simulink subsystem "tcp_trace_simscape_ref_subsys"  (R2022b)
settings: Solver=VariableStepAuto  StartTime=0.0  StopTime=10.0  RelTol=1e-3
undefined symbols (not defined in the file): param_vis
libraries: nesl_utility x300, sm_lib x200
(part 2 of 3)

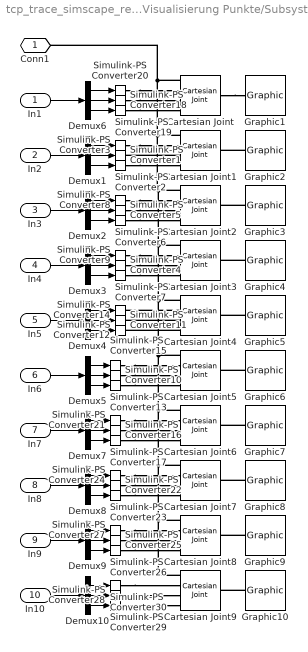
== system tcp_trace_simscape_ref_subsys/Visualisierung Punkte/Subsystem3 ==
  In1 : Inport
  In2 : Inport  Port=2
  In3 : Inport  Port=3
  In4 : Inport  Port=4
  In5 : Inport  Port=5
  In6 : Inport  Port=6
  In7 : Inport  Port=7
  In8 : Inport  Port=8
  In9 : Inport  Port=9
  In10 : Inport  Port=10
  Cartesian Joint{,1..9} (10 alike) : sm_lib/Joints/Cartesian Joint  JointMode=Normal  SenseConstraintForce=off  SenseConstraintForceX=off  SenseConstraintForceY=off  SenseConstraintForceZ=off  SenseConstraintTorque=off  SenseConstraintTorqueX=off  SenseConstraintTorqueY=off  SenseConstraintTorqueZ=off  SenseTotalForce=off  SenseTotalForceX=off  SenseTotalForceY=off  SenseTotalForceZ=off  SenseTotalTorque=off  SenseTotalTorqueX=off  SenseTotalTorqueY=off  SenseTotalTorqueZ=off  CompositeWrenchDir=FollowerOnBase  CompositeWrenchFrame=BaseFrame  PxEquilibriumPosition=0  PxEquilibriumPositionUnits=m  PxSpringStiffness=0  PxSpringStiffnessUnits=N/m  PxDampingCoefficient=0  PxDampingCoefficientUnits=N/(m/s)  PxTorqueActuationMode=ComputedTorque  PxMotionActuationMode=InputMotion  PxSensePosition=off  PxSenseVelocity=off  PxSenseAcceleration=off  PxSenseTorqueForce=off  PxSenseLowerLimitTorqueForce=off  PxSenseUpperLimitTorqueForce=off  PxLowerLimitSpecify=off  PxLowerLimitBound=-1  PxLowerLimitBoundUnits=m  PxLowerLimitStiffness=1e6  PxLowerLimitStiffnessUnits=N/m  PxLowerLimitDamping=1e3  PxLowerLimitDampingUnits=N/(m/s)  PxLowerLimitTransitionRegionWidth=1e-4  PxLowerLimitTransitionRegionWidthUnits=m  PxUpperLimitSpecify=off  PxUpperLimitBound=1  PxUpperLimitBoundUnits=m  PxUpperLimitStiffness=1e6  PxUpperLimitStiffnessUnits=N/m  PxUpperLimitDamping=1e3  PxUpperLimitDampingUnits=N/(m/s)  PxUpperLimitTransitionRegionWidth=1e-4  PxUpperLimitTransitionRegionWidthUnits=m  PxPositionTargetSpecify=off  PxPositionTargetPriority=High  PxPositionTargetValue=0  PxPositionTargetValueUnits=m  PxVelocityTargetSpecify=off  PxVelocityTargetPriority=High  PxVelocityTargetValue=0  PxVelocityTargetValueUnits=m/s  PyEquilibriumPosition=0  PyEquilibriumPositionUnits=m  PySpringStiffness=0  PySpringStiffnessUnits=N/m  PyDampingCoefficient=0  PyDampingCoefficientUnits=N/(m/s)  PyTorqueActuationMode=ComputedTorque  PyMotionActuationMode=InputMotion  PySensePosition=off  PySenseVelocity=off  PySenseAcceleration=off  PySenseTorqueForce=off  PySenseLowerLimitTorqueForce=off  PySenseUpperLimitTorqueForce=off  PyLowerLimitSpecify=off  PyLowerLimitBound=-1  PyLowerLimitBoundUnits=m  PyLowerLimitStiffness=1e6  PyLowerLimitStiffnessUnits=N/m  PyLowerLimitDamping=1e3  PyLowerLimitDampingUnits=N/(m/s)  PyLowerLimitTransitionRegionWidth=1e-4  PyLowerLimitTransitionRegionWidthUnits=m  PyUpperLimitSpecify=off  PyUpperLimitBound=1  PyUpperLimitBoundUnits=m  PyUpperLimitStiffness=1e6  PyUpperLimitStiffnessUnits=N/m  PyUpperLimitDamping=1e3  PyUpperLimitDampingUnits=N/(m/s)  PyUpperLimitTransitionRegionWidth=1e-4  PyUpperLimitTransitionRegionWidthUnits=m  PyPositionTargetSpecify=off  PyPositionTargetPriority=High  PyPositionTargetValue=0  PyPositionTargetValueUnits=m  PyVelocityTargetSpecify=off  PyVelocityTargetPriority=High  PyVelocityTargetValue=0  PyVelocityTargetValueUnits=m/s  PzEquilibriumPosition=0  PzEquilibriumPositionUnits=m  PzSpringStiffness=0  PzSpringStiffnessUnits=N/m  PzDampingCoefficient=0  PzDampingCoefficientUnits=N/(m/s)  PzTorqueActuationMode=ComputedTorque  PzMotionActuationMode=InputMotion  PzSensePosition=off  PzSenseVelocity=off  PzSenseAcceleration=off  PzSenseTorqueForce=off  PzSenseLowerLimitTorqueForce=off  PzSenseUpperLimitTorqueForce=off  PzLowerLimitSpecify=off  PzLowerLimitBound=-1  PzLowerLimitBoundUnits=m  PzLowerLimitStiffness=1e6  PzLowerLimitStiffnessUnits=N/m  PzLowerLimitDamping=1e3  PzLowerLimitDampingUnits=N/(m/s)  PzLowerLimitTransitionRegionWidth=1e-4  PzLowerLimitTransitionRegionWidthUnits=m  PzUpperLimitSpecify=off  PzUpperLimitBound=1  PzUpperLimitBoundUnits=m  PzUpperLimitStiffness=1e6  PzUpperLimitStiffnessUnits=N/m  PzUpperLimitDamping=1e3  PzUpperLimitDampingUnits=N/(m/s)  PzUpperLimitTransitionRegionWidth=1e-4  PzUpperLimitTransitionRegionWidthUnits=m  PzPositionTargetSpecify=off  PzPositionTargetPriority=High  PzPositionTargetValue=0  PzPositionTargetValueUnits=m  PzVelocityTargetSpecify=off  PzVelocityTargetPriority=High  PzVelocityTargetValue=0  PzVelocityTargetValueUnits=m/s
  Demux{1..10} (10 alike) : Demux  Outputs=3
  Graphic{1..10} (10 alike) : sm_lib/Body Elements/Graphic  GraphicType=Marker  MarkerShape=Sphere  MarkerSize=param_vis.vis_point.pix  GraphicVisPropType=SimpleVisualProperties  GraphicDiffuseColor=param_vis.vis_point.col  GraphicSpecularColor=[0.5 0.5 0.5 1.0]  GraphicAmbientColor=[0.15 0.15 0.15 1.0]  GraphicEmissiveColor=[0.0 0.0 0.0 1.0]  GraphicShininess=75  GraphicOpacity=param_vis.vis_point.opa
  Simulink-PS Converter{1..30} (30 alike) : nesl_utility/Simulink-PS Converter  PhysicalDomain=network_engine_domain  SubClassName=ps_input  LeftPortType=input  RightPortType=output  PseudoPeriodic=off  Frequencies=[]  NoiseDistribution=none  NoiseParameters=[]  Unit=1  AffineConversion=off  FilteringAndDerivatives=zero  SimscapeFilterOrder=2  InputFilterTimeConstant=0.001  UdotUserProvided=0
  Conn1 : PMIOPort  Side=Left
  wires:
  Demux10/3 -> Simulink-PS Converter29/1
  Demux10/2 -> Simulink-PS Converter28/1
  Demux10/1 -> Simulink-PS Converter30/1
  Demux9/3 -> Simulink-PS Converter26/1
  Demux9/2 -> Simulink-PS Converter25/1
  Demux9/1 -> Simulink-PS Converter27/1
  Demux8/3 -> Simulink-PS Converter23/1
  Demux8/2 -> Simulink-PS Converter22/1
  Demux8/1 -> Simulink-PS Converter24/1
  Demux7/3 -> Simulink-PS Converter17/1
  Demux7/2 -> Simulink-PS Converter16/1
  Demux7/1 -> Simulink-PS Converter21/1
  Demux5/3 -> Simulink-PS Converter13/1
  Demux5/2 -> Simulink-PS Converter10/1
  Demux5/1 -> Simulink-PS Converter15/1
  Demux3/2 -> Simulink-PS Converter4/1
  Demux3/1 -> Simulink-PS Converter9/1
  Demux3/3 -> Simulink-PS Converter7/1
  Demux2/3 -> Simulink-PS Converter6/1
  Demux2/2 -> Simulink-PS Converter5/1
  Demux2/1 -> Simulink-PS Converter8/1
  Demux1/3 -> Simulink-PS Converter2/1
  Demux1/2 -> Simulink-PS Converter1/1
  Demux4/3 -> Simulink-PS Converter12/1
  Demux4/1 -> Simulink-PS Converter14/1
  Demux4/2 -> Simulink-PS Converter11/1
  Demux1/1 -> Simulink-PS Converter3/1
  Demux6/2 -> Simulink-PS Converter18/1
  Demux6/1 -> Simulink-PS Converter20/1
  In8/1 -> Demux8/1
  In9/1 -> Demux9/1
  In1/1 -> Demux6/1
  In3/1 -> Demux2/1
  Demux6/3 -> Simulink-PS Converter19/1
  In4/1 -> Demux3/1
  In5/1 -> Demux4/1
  In2/1 -> Demux1/1
  In10/1 -> Demux10/1
  In6/1 -> Demux5/1
  In7/1 -> Demux7/1
  connections:
  Simulink-PS Converter7/RConn1 -- Cartesian Joint3/LConn4
  Simulink-PS Converter4/RConn1 -- Cartesian Joint3/LConn3
  Simulink-PS Converter9/RConn1 -- Cartesian Joint3/LConn2
  Simulink-PS Converter29/RConn1 -- Cartesian Joint9/LConn4
  Simulink-PS Converter28/RConn1 -- Cartesian Joint9/LConn3
  Simulink-PS Converter30/RConn1 -- Cartesian Joint9/LConn2
  Simulink-PS Converter26/RConn1 -- Cartesian Joint8/LConn4
  Simulink-PS Converter25/RConn1 -- Cartesian Joint8/LConn3
  Simulink-PS Converter27/RConn1 -- Cartesian Joint8/LConn2
  Simulink-PS Converter23/RConn1 -- Cartesian Joint7/LConn4
  Simulink-PS Converter22/RConn1 -- Cartesian Joint7/LConn3
  Simulink-PS Converter24/RConn1 -- Cartesian Joint7/LConn2
  Simulink-PS Converter17/RConn1 -- Cartesian Joint6/LConn4
  Simulink-PS Converter16/RConn1 -- Cartesian Joint6/LConn3
  Simulink-PS Converter21/RConn1 -- Cartesian Joint6/LConn2
  Simulink-PS Converter13/RConn1 -- Cartesian Joint5/LConn4
  Simulink-PS Converter10/RConn1 -- Cartesian Joint5/LConn3
  Simulink-PS Converter15/RConn1 -- Cartesian Joint5/LConn2
  Simulink-PS Converter2/RConn1 -- Cartesian Joint1/LConn4
  Cartesian Joint1/LConn3 -- Simulink-PS Converter1/RConn1
  Simulink-PS Converter3/RConn1 -- Cartesian Joint1/LConn2
  Cartesian Joint4/LConn3 -- Simulink-PS Converter11/RConn1
  Cartesian Joint4/LConn2 -- Simulink-PS Converter14/RConn1
  Cartesian Joint4/LConn4 -- Simulink-PS Converter12/RConn1
  Simulink-PS Converter5/RConn1 -- Cartesian Joint2/LConn3
  Simulink-PS Converter8/RConn1 -- Cartesian Joint2/LConn2
  Simulink-PS Converter6/RConn1 -- Cartesian Joint2/LConn4
  Simulink-PS Converter20/RConn1 -- Cartesian Joint/LConn2
  Simulink-PS Converter18/RConn1 -- Cartesian Joint/LConn3
  Graphic10/RConn1 -- Cartesian Joint9/RConn1
  Graphic5/RConn1 -- Cartesian Joint4/RConn1
  Graphic2/RConn1 -- Cartesian Joint1/RConn1
  Graphic9/RConn1 -- Cartesian Joint8/RConn1
  Graphic6/RConn1 -- Cartesian Joint5/RConn1
  Graphic8/RConn1 -- Cartesian Joint7/RConn1
  Graphic7/RConn1 -- Cartesian Joint6/RConn1
  Conn1/RConn1 -- Cartesian Joint/LConn1 -- Cartesian Joint1/LConn1 -- Cartesian Joint2/LConn1 -- Cartesian Joint3/LConn1 -- Cartesian Joint4/LConn1 -- Cartesian Joint5/LConn1 -- Cartesian Joint6/LConn1 -- Cartesian Joint7/LConn1 -- Cartesian Joint9/LConn1 -- Cartesian Joint8/LConn1
  Graphic3/RConn1 -- Cartesian Joint2/RConn1
  Cartesian Joint/RConn1 -- Graphic1/RConn1
  Graphic4/RConn1 -- Cartesian Joint3/RConn1
  Simulink-PS Converter19/RConn1 -- Cartesian Joint/LConn4

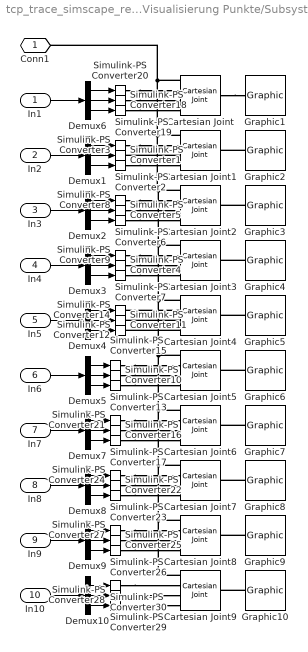
== system tcp_trace_simscape_ref_subsys/Visualisierung Punkte/Subsystem4 ==
  In1 : Inport
  In2 : Inport  Port=2
  In3 : Inport  Port=3
  In4 : Inport  Port=4
  In5 : Inport  Port=5
  In6 : Inport  Port=6
  In7 : Inport  Port=7
  In8 : Inport  Port=8
  In9 : Inport  Port=9
  In10 : Inport  Port=10
  Cartesian Joint{,1..9} (10 alike) : sm_lib/Joints/Cartesian Joint  JointMode=Normal  SenseConstraintForce=off  SenseConstraintForceX=off  SenseConstraintForceY=off  SenseConstraintForceZ=off  SenseConstraintTorque=off  SenseConstraintTorqueX=off  SenseConstraintTorqueY=off  SenseConstraintTorqueZ=off  SenseTotalForce=off  SenseTotalForceX=off  SenseTotalForceY=off  SenseTotalForceZ=off  SenseTotalTorque=off  SenseTotalTorqueX=off  SenseTotalTorqueY=off  SenseTotalTorqueZ=off  CompositeWrenchDir=FollowerOnBase  CompositeWrenchFrame=BaseFrame  PxEquilibriumPosition=0  PxEquilibriumPositionUnits=m  PxSpringStiffness=0  PxSpringStiffnessUnits=N/m  PxDampingCoefficient=0  PxDampingCoefficientUnits=N/(m/s)  PxTorqueActuationMode=ComputedTorque  PxMotionActuationMode=InputMotion  PxSensePosition=off  PxSenseVelocity=off  PxSenseAcceleration=off  PxSenseTorqueForce=off  PxSenseLowerLimitTorqueForce=off  PxSenseUpperLimitTorqueForce=off  PxLowerLimitSpecify=off  PxLowerLimitBound=-1  PxLowerLimitBoundUnits=m  PxLowerLimitStiffness=1e6  PxLowerLimitStiffnessUnits=N/m  PxLowerLimitDamping=1e3  PxLowerLimitDampingUnits=N/(m/s)  PxLowerLimitTransitionRegionWidth=1e-4  PxLowerLimitTransitionRegionWidthUnits=m  PxUpperLimitSpecify=off  PxUpperLimitBound=1  PxUpperLimitBoundUnits=m  PxUpperLimitStiffness=1e6  PxUpperLimitStiffnessUnits=N/m  PxUpperLimitDamping=1e3  PxUpperLimitDampingUnits=N/(m/s)  PxUpperLimitTransitionRegionWidth=1e-4  PxUpperLimitTransitionRegionWidthUnits=m  PxPositionTargetSpecify=off  PxPositionTargetPriority=High  PxPositionTargetValue=0  PxPositionTargetValueUnits=m  PxVelocityTargetSpecify=off  PxVelocityTargetPriority=High  PxVelocityTargetValue=0  PxVelocityTargetValueUnits=m/s  PyEquilibriumPosition=0  PyEquilibriumPositionUnits=m  PySpringStiffness=0  PySpringStiffnessUnits=N/m  PyDampingCoefficient=0  PyDampingCoefficientUnits=N/(m/s)  PyTorqueActuationMode=ComputedTorque  PyMotionActuationMode=InputMotion  PySensePosition=off  PySenseVelocity=off  PySenseAcceleration=off  PySenseTorqueForce=off  PySenseLowerLimitTorqueForce=off  PySenseUpperLimitTorqueForce=off  PyLowerLimitSpecify=off  PyLowerLimitBound=-1  PyLowerLimitBoundUnits=m  PyLowerLimitStiffness=1e6  PyLowerLimitStiffnessUnits=N/m  PyLowerLimitDamping=1e3  PyLowerLimitDampingUnits=N/(m/s)  PyLowerLimitTransitionRegionWidth=1e-4  PyLowerLimitTransitionRegionWidthUnits=m  PyUpperLimitSpecify=off  PyUpperLimitBound=1  PyUpperLimitBoundUnits=m  PyUpperLimitStiffness=1e6  PyUpperLimitStiffnessUnits=N/m  PyUpperLimitDamping=1e3  PyUpperLimitDampingUnits=N/(m/s)  PyUpperLimitTransitionRegionWidth=1e-4  PyUpperLimitTransitionRegionWidthUnits=m  PyPositionTargetSpecify=off  PyPositionTargetPriority=High  PyPositionTargetValue=0  PyPositionTargetValueUnits=m  PyVelocityTargetSpecify=off  PyVelocityTargetPriority=High  PyVelocityTargetValue=0  PyVelocityTargetValueUnits=m/s  PzEquilibriumPosition=0  PzEquilibriumPositionUnits=m  PzSpringStiffness=0  PzSpringStiffnessUnits=N/m  PzDampingCoefficient=0  PzDampingCoefficientUnits=N/(m/s)  PzTorqueActuationMode=ComputedTorque  PzMotionActuationMode=InputMotion  PzSensePosition=off  PzSenseVelocity=off  PzSenseAcceleration=off  PzSenseTorqueForce=off  PzSenseLowerLimitTorqueForce=off  PzSenseUpperLimitTorqueForce=off  PzLowerLimitSpecify=off  PzLowerLimitBound=-1  PzLowerLimitBoundUnits=m  PzLowerLimitStiffness=1e6  PzLowerLimitStiffnessUnits=N/m  PzLowerLimitDamping=1e3  PzLowerLimitDampingUnits=N/(m/s)  PzLowerLimitTransitionRegionWidth=1e-4  PzLowerLimitTransitionRegionWidthUnits=m  PzUpperLimitSpecify=off  PzUpperLimitBound=1  PzUpperLimitBoundUnits=m  PzUpperLimitStiffness=1e6  PzUpperLimitStiffnessUnits=N/m  PzUpperLimitDamping=1e3  PzUpperLimitDampingUnits=N/(m/s)  PzUpperLimitTransitionRegionWidth=1e-4  PzUpperLimitTransitionRegionWidthUnits=m  PzPositionTargetSpecify=off  PzPositionTargetPriority=High  PzPositionTargetValue=0  PzPositionTargetValueUnits=m  PzVelocityTargetSpecify=off  PzVelocityTargetPriority=High  PzVelocityTargetValue=0  PzVelocityTargetValueUnits=m/s
  Demux{1..10} (10 alike) : Demux  Outputs=3
  Graphic{1..10} (10 alike) : sm_lib/Body Elements/Graphic  GraphicType=Marker  MarkerShape=Sphere  MarkerSize=param_vis.vis_point.pix  GraphicVisPropType=SimpleVisualProperties  GraphicDiffuseColor=param_vis.vis_point.col  GraphicSpecularColor=[0.5 0.5 0.5 1.0]  GraphicAmbientColor=[0.15 0.15 0.15 1.0]  GraphicEmissiveColor=[0.0 0.0 0.0 1.0]  GraphicShininess=75  GraphicOpacity=param_vis.vis_point.opa
  Simulink-PS Converter{1..30} (30 alike) : nesl_utility/Simulink-PS Converter  PhysicalDomain=network_engine_domain  SubClassName=ps_input  LeftPortType=input  RightPortType=output  PseudoPeriodic=off  Frequencies=[]  NoiseDistribution=none  NoiseParameters=[]  Unit=1  AffineConversion=off  FilteringAndDerivatives=zero  SimscapeFilterOrder=2  InputFilterTimeConstant=0.001  UdotUserProvided=0
  Conn1 : PMIOPort  Side=Left
  wires:
  In7/1 -> Demux7/1
  In6/1 -> Demux5/1
  In10/1 -> Demux10/1
  In2/1 -> Demux1/1
  In5/1 -> Demux4/1
  In4/1 -> Demux3/1
  Demux6/3 -> Simulink-PS Converter19/1
  In3/1 -> Demux2/1
  In1/1 -> Demux6/1
  In9/1 -> Demux9/1
  In8/1 -> Demux8/1
  Demux6/1 -> Simulink-PS Converter20/1
  Demux6/2 -> Simulink-PS Converter18/1
  Demux1/1 -> Simulink-PS Converter3/1
  Demux4/2 -> Simulink-PS Converter11/1
  Demux4/1 -> Simulink-PS Converter14/1
  Demux4/3 -> Simulink-PS Converter12/1
  Demux1/2 -> Simulink-PS Converter1/1
  Demux1/3 -> Simulink-PS Converter2/1
  Demux2/1 -> Simulink-PS Converter8/1
  Demux2/2 -> Simulink-PS Converter5/1
  Demux2/3 -> Simulink-PS Converter6/1
  Demux3/3 -> Simulink-PS Converter7/1
  Demux3/1 -> Simulink-PS Converter9/1
  Demux3/2 -> Simulink-PS Converter4/1
  Demux5/1 -> Simulink-PS Converter15/1
  Demux5/2 -> Simulink-PS Converter10/1
  Demux5/3 -> Simulink-PS Converter13/1
  Demux7/1 -> Simulink-PS Converter21/1
  Demux7/2 -> Simulink-PS Converter16/1
  Demux7/3 -> Simulink-PS Converter17/1
  Demux8/1 -> Simulink-PS Converter24/1
  Demux8/2 -> Simulink-PS Converter22/1
  Demux8/3 -> Simulink-PS Converter23/1
  Demux9/1 -> Simulink-PS Converter27/1
  Demux9/2 -> Simulink-PS Converter25/1
  Demux9/3 -> Simulink-PS Converter26/1
  Demux10/1 -> Simulink-PS Converter30/1
  Demux10/2 -> Simulink-PS Converter28/1
  Demux10/3 -> Simulink-PS Converter29/1
  connections:
  Simulink-PS Converter19/RConn1 -- Cartesian Joint/LConn4
  Graphic4/RConn1 -- Cartesian Joint3/RConn1
  Cartesian Joint/RConn1 -- Graphic1/RConn1
  Graphic3/RConn1 -- Cartesian Joint2/RConn1
  Cartesian Joint8/LConn1 -- Cartesian Joint9/LConn1 -- Cartesian Joint7/LConn1 -- Cartesian Joint6/LConn1 -- Cartesian Joint5/LConn1 -- Cartesian Joint4/LConn1 -- Cartesian Joint3/LConn1 -- Cartesian Joint2/LConn1 -- Cartesian Joint1/LConn1 -- Cartesian Joint/LConn1 -- Conn1/RConn1
  Graphic7/RConn1 -- Cartesian Joint6/RConn1
  Graphic8/RConn1 -- Cartesian Joint7/RConn1
  Graphic6/RConn1 -- Cartesian Joint5/RConn1
  Graphic9/RConn1 -- Cartesian Joint8/RConn1
  Graphic2/RConn1 -- Cartesian Joint1/RConn1
  Graphic5/RConn1 -- Cartesian Joint4/RConn1
  Graphic10/RConn1 -- Cartesian Joint9/RConn1
  Simulink-PS Converter18/RConn1 -- Cartesian Joint/LConn3
  Simulink-PS Converter20/RConn1 -- Cartesian Joint/LConn2
  Simulink-PS Converter6/RConn1 -- Cartesian Joint2/LConn4
  Simulink-PS Converter8/RConn1 -- Cartesian Joint2/LConn2
  Simulink-PS Converter5/RConn1 -- Cartesian Joint2/LConn3
  Cartesian Joint4/LConn4 -- Simulink-PS Converter12/RConn1
  Cartesian Joint4/LConn2 -- Simulink-PS Converter14/RConn1
  Cartesian Joint4/LConn3 -- Simulink-PS Converter11/RConn1
  Simulink-PS Converter3/RConn1 -- Cartesian Joint1/LConn2
  Cartesian Joint1/LConn3 -- Simulink-PS Converter1/RConn1
  Simulink-PS Converter2/RConn1 -- Cartesian Joint1/LConn4
  Simulink-PS Converter15/RConn1 -- Cartesian Joint5/LConn2
  Simulink-PS Converter10/RConn1 -- Cartesian Joint5/LConn3
  Simulink-PS Converter13/RConn1 -- Cartesian Joint5/LConn4
  Simulink-PS Converter21/RConn1 -- Cartesian Joint6/LConn2
  Simulink-PS Converter16/RConn1 -- Cartesian Joint6/LConn3
  Simulink-PS Converter17/RConn1 -- Cartesian Joint6/LConn4
  Simulink-PS Converter24/RConn1 -- Cartesian Joint7/LConn2
  Simulink-PS Converter22/RConn1 -- Cartesian Joint7/LConn3
  Simulink-PS Converter23/RConn1 -- Cartesian Joint7/LConn4
  Simulink-PS Converter27/RConn1 -- Cartesian Joint8/LConn2
  Simulink-PS Converter25/RConn1 -- Cartesian Joint8/LConn3
  Simulink-PS Converter26/RConn1 -- Cartesian Joint8/LConn4
  Simulink-PS Converter30/RConn1 -- Cartesian Joint9/LConn2
  Simulink-PS Converter28/RConn1 -- Cartesian Joint9/LConn3
  Simulink-PS Converter29/RConn1 -- Cartesian Joint9/LConn4
  Simulink-PS Converter9/RConn1 -- Cartesian Joint3/LConn2
  Simulink-PS Converter4/RConn1 -- Cartesian Joint3/LConn3
  Simulink-PS Converter7/RConn1 -- Cartesian Joint3/LConn4

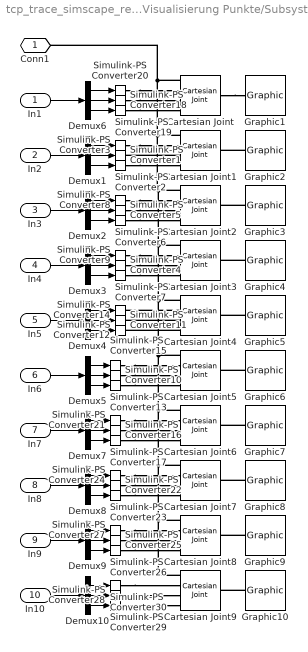
== system tcp_trace_simscape_ref_subsys/Visualisierung Punkte/Subsystem5 ==
  In1 : Inport
  In2 : Inport  Port=2
  In3 : Inport  Port=3
  In4 : Inport  Port=4
  In5 : Inport  Port=5
  In6 : Inport  Port=6
  In7 : Inport  Port=7
  In8 : Inport  Port=8
  In9 : Inport  Port=9
  In10 : Inport  Port=10
  Cartesian Joint{,1..9} (10 alike) : sm_lib/Joints/Cartesian Joint  JointMode=Normal  SenseConstraintForce=off  SenseConstraintForceX=off  SenseConstraintForceY=off  SenseConstraintForceZ=off  SenseConstraintTorque=off  SenseConstraintTorqueX=off  SenseConstraintTorqueY=off  SenseConstraintTorqueZ=off  SenseTotalForce=off  SenseTotalForceX=off  SenseTotalForceY=off  SenseTotalForceZ=off  SenseTotalTorque=off  SenseTotalTorqueX=off  SenseTotalTorqueY=off  SenseTotalTorqueZ=off  CompositeWrenchDir=FollowerOnBase  CompositeWrenchFrame=BaseFrame  PxEquilibriumPosition=0  PxEquilibriumPositionUnits=m  PxSpringStiffness=0  PxSpringStiffnessUnits=N/m  PxDampingCoefficient=0  PxDampingCoefficientUnits=N/(m/s)  PxTorqueActuationMode=ComputedTorque  PxMotionActuationMode=InputMotion  PxSensePosition=off  PxSenseVelocity=off  PxSenseAcceleration=off  PxSenseTorqueForce=off  PxSenseLowerLimitTorqueForce=off  PxSenseUpperLimitTorqueForce=off  PxLowerLimitSpecify=off  PxLowerLimitBound=-1  PxLowerLimitBoundUnits=m  PxLowerLimitStiffness=1e6  PxLowerLimitStiffnessUnits=N/m  PxLowerLimitDamping=1e3  PxLowerLimitDampingUnits=N/(m/s)  PxLowerLimitTransitionRegionWidth=1e-4  PxLowerLimitTransitionRegionWidthUnits=m  PxUpperLimitSpecify=off  PxUpperLimitBound=1  PxUpperLimitBoundUnits=m  PxUpperLimitStiffness=1e6  PxUpperLimitStiffnessUnits=N/m  PxUpperLimitDamping=1e3  PxUpperLimitDampingUnits=N/(m/s)  PxUpperLimitTransitionRegionWidth=1e-4  PxUpperLimitTransitionRegionWidthUnits=m  PxPositionTargetSpecify=off  PxPositionTargetPriority=High  PxPositionTargetValue=0  PxPositionTargetValueUnits=m  PxVelocityTargetSpecify=off  PxVelocityTargetPriority=High  PxVelocityTargetValue=0  PxVelocityTargetValueUnits=m/s  PyEquilibriumPosition=0  PyEquilibriumPositionUnits=m  PySpringStiffness=0  PySpringStiffnessUnits=N/m  PyDampingCoefficient=0  PyDampingCoefficientUnits=N/(m/s)  PyTorqueActuationMode=ComputedTorque  PyMotionActuationMode=InputMotion  PySensePosition=off  PySenseVelocity=off  PySenseAcceleration=off  PySenseTorqueForce=off  PySenseLowerLimitTorqueForce=off  PySenseUpperLimitTorqueForce=off  PyLowerLimitSpecify=off  PyLowerLimitBound=-1  PyLowerLimitBoundUnits=m  PyLowerLimitStiffness=1e6  PyLowerLimitStiffnessUnits=N/m  PyLowerLimitDamping=1e3  PyLowerLimitDampingUnits=N/(m/s)  PyLowerLimitTransitionRegionWidth=1e-4  PyLowerLimitTransitionRegionWidthUnits=m  PyUpperLimitSpecify=off  PyUpperLimitBound=1  PyUpperLimitBoundUnits=m  PyUpperLimitStiffness=1e6  PyUpperLimitStiffnessUnits=N/m  PyUpperLimitDamping=1e3  PyUpperLimitDampingUnits=N/(m/s)  PyUpperLimitTransitionRegionWidth=1e-4  PyUpperLimitTransitionRegionWidthUnits=m  PyPositionTargetSpecify=off  PyPositionTargetPriority=High  PyPositionTargetValue=0  PyPositionTargetValueUnits=m  PyVelocityTargetSpecify=off  PyVelocityTargetPriority=High  PyVelocityTargetValue=0  PyVelocityTargetValueUnits=m/s  PzEquilibriumPosition=0  PzEquilibriumPositionUnits=m  PzSpringStiffness=0  PzSpringStiffnessUnits=N/m  PzDampingCoefficient=0  PzDampingCoefficientUnits=N/(m/s)  PzTorqueActuationMode=ComputedTorque  PzMotionActuationMode=InputMotion  PzSensePosition=off  PzSenseVelocity=off  PzSenseAcceleration=off  PzSenseTorqueForce=off  PzSenseLowerLimitTorqueForce=off  PzSenseUpperLimitTorqueForce=off  PzLowerLimitSpecify=off  PzLowerLimitBound=-1  PzLowerLimitBoundUnits=m  PzLowerLimitStiffness=1e6  PzLowerLimitStiffnessUnits=N/m  PzLowerLimitDamping=1e3  PzLowerLimitDampingUnits=N/(m/s)  PzLowerLimitTransitionRegionWidth=1e-4  PzLowerLimitTransitionRegionWidthUnits=m  PzUpperLimitSpecify=off  PzUpperLimitBound=1  PzUpperLimitBoundUnits=m  PzUpperLimitStiffness=1e6  PzUpperLimitStiffnessUnits=N/m  PzUpperLimitDamping=1e3  PzUpperLimitDampingUnits=N/(m/s)  PzUpperLimitTransitionRegionWidth=1e-4  PzUpperLimitTransitionRegionWidthUnits=m  PzPositionTargetSpecify=off  PzPositionTargetPriority=High  PzPositionTargetValue=0  PzPositionTargetValueUnits=m  PzVelocityTargetSpecify=off  PzVelocityTargetPriority=High  PzVelocityTargetValue=0  PzVelocityTargetValueUnits=m/s
  Demux{1..10} (10 alike) : Demux  Outputs=3
  Graphic{1..10} (10 alike) : sm_lib/Body Elements/Graphic  GraphicType=Marker  MarkerShape=Sphere  MarkerSize=param_vis.vis_point.pix  GraphicVisPropType=SimpleVisualProperties  GraphicDiffuseColor=param_vis.vis_point.col  GraphicSpecularColor=[0.5 0.5 0.5 1.0]  GraphicAmbientColor=[0.15 0.15 0.15 1.0]  GraphicEmissiveColor=[0.0 0.0 0.0 1.0]  GraphicShininess=75  GraphicOpacity=param_vis.vis_point.opa
  Simulink-PS Converter{1..30} (30 alike) : nesl_utility/Simulink-PS Converter  PhysicalDomain=network_engine_domain  SubClassName=ps_input  LeftPortType=input  RightPortType=output  PseudoPeriodic=off  Frequencies=[]  NoiseDistribution=none  NoiseParameters=[]  Unit=1  AffineConversion=off  FilteringAndDerivatives=zero  SimscapeFilterOrder=2  InputFilterTimeConstant=0.001  UdotUserProvided=0
  Conn1 : PMIOPort  Side=Left
  wires:
  Demux10/3 -> Simulink-PS Converter29/1
  Demux10/2 -> Simulink-PS Converter28/1
  Demux10/1 -> Simulink-PS Converter30/1
  Demux9/3 -> Simulink-PS Converter26/1
  Demux9/2 -> Simulink-PS Converter25/1
  Demux9/1 -> Simulink-PS Converter27/1
  Demux8/3 -> Simulink-PS Converter23/1
  Demux8/2 -> Simulink-PS Converter22/1
  Demux8/1 -> Simulink-PS Converter24/1
  Demux7/3 -> Simulink-PS Converter17/1
  Demux7/2 -> Simulink-PS Converter16/1
  Demux7/1 -> Simulink-PS Converter21/1
  Demux5/3 -> Simulink-PS Converter13/1
  Demux5/2 -> Simulink-PS Converter10/1
  Demux5/1 -> Simulink-PS Converter15/1
  Demux3/2 -> Simulink-PS Converter4/1
  Demux3/1 -> Simulink-PS Converter9/1
  Demux3/3 -> Simulink-PS Converter7/1
  Demux2/3 -> Simulink-PS Converter6/1
  Demux2/2 -> Simulink-PS Converter5/1
  Demux2/1 -> Simulink-PS Converter8/1
  Demux1/3 -> Simulink-PS Converter2/1
  Demux1/2 -> Simulink-PS Converter1/1
  Demux4/3 -> Simulink-PS Converter12/1
  Demux4/1 -> Simulink-PS Converter14/1
  Demux4/2 -> Simulink-PS Converter11/1
  Demux1/1 -> Simulink-PS Converter3/1
  Demux6/2 -> Simulink-PS Converter18/1
  Demux6/1 -> Simulink-PS Converter20/1
  In8/1 -> Demux8/1
  In9/1 -> Demux9/1
  In1/1 -> Demux6/1
  In3/1 -> Demux2/1
  Demux6/3 -> Simulink-PS Converter19/1
  In4/1 -> Demux3/1
  In5/1 -> Demux4/1
  In2/1 -> Demux1/1
  In10/1 -> Demux10/1
  In6/1 -> Demux5/1
  In7/1 -> Demux7/1
  connections:
  Simulink-PS Converter7/RConn1 -- Cartesian Joint3/LConn4
  Simulink-PS Converter4/RConn1 -- Cartesian Joint3/LConn3
  Simulink-PS Converter9/RConn1 -- Cartesian Joint3/LConn2
  Simulink-PS Converter29/RConn1 -- Cartesian Joint9/LConn4
  Simulink-PS Converter28/RConn1 -- Cartesian Joint9/LConn3
  Simulink-PS Converter30/RConn1 -- Cartesian Joint9/LConn2
  Simulink-PS Converter26/RConn1 -- Cartesian Joint8/LConn4
  Simulink-PS Converter25/RConn1 -- Cartesian Joint8/LConn3
  Simulink-PS Converter27/RConn1 -- Cartesian Joint8/LConn2
  Simulink-PS Converter23/RConn1 -- Cartesian Joint7/LConn4
  Simulink-PS Converter22/RConn1 -- Cartesian Joint7/LConn3
  Simulink-PS Converter24/RConn1 -- Cartesian Joint7/LConn2
  Simulink-PS Converter17/RConn1 -- Cartesian Joint6/LConn4
  Simulink-PS Converter16/RConn1 -- Cartesian Joint6/LConn3
  Simulink-PS Converter21/RConn1 -- Cartesian Joint6/LConn2
  Simulink-PS Converter13/RConn1 -- Cartesian Joint5/LConn4
  Simulink-PS Converter10/RConn1 -- Cartesian Joint5/LConn3
  Simulink-PS Converter15/RConn1 -- Cartesian Joint5/LConn2
  Simulink-PS Converter2/RConn1 -- Cartesian Joint1/LConn4
  Cartesian Joint1/LConn3 -- Simulink-PS Converter1/RConn1
  Simulink-PS Converter3/RConn1 -- Cartesian Joint1/LConn2
  Cartesian Joint4/LConn3 -- Simulink-PS Converter11/RConn1
  Cartesian Joint4/LConn2 -- Simulink-PS Converter14/RConn1
  Cartesian Joint4/LConn4 -- Simulink-PS Converter12/RConn1
  Simulink-PS Converter5/RConn1 -- Cartesian Joint2/LConn3
  Simulink-PS Converter8/RConn1 -- Cartesian Joint2/LConn2
  Simulink-PS Converter6/RConn1 -- Cartesian Joint2/LConn4
  Simulink-PS Converter20/RConn1 -- Cartesian Joint/LConn2
  Simulink-PS Converter18/RConn1 -- Cartesian Joint/LConn3
  Graphic10/RConn1 -- Cartesian Joint9/RConn1
  Graphic5/RConn1 -- Cartesian Joint4/RConn1
  Graphic2/RConn1 -- Cartesian Joint1/RConn1
  Graphic9/RConn1 -- Cartesian Joint8/RConn1
  Graphic6/RConn1 -- Cartesian Joint5/RConn1
  Graphic8/RConn1 -- Cartesian Joint7/RConn1
  Graphic7/RConn1 -- Cartesian Joint6/RConn1
  Conn1/RConn1 -- Cartesian Joint/LConn1 -- Cartesian Joint1/LConn1 -- Cartesian Joint2/LConn1 -- Cartesian Joint3/LConn1 -- Cartesian Joint4/LConn1 -- Cartesian Joint5/LConn1 -- Cartesian Joint6/LConn1 -- Cartesian Joint7/LConn1 -- Cartesian Joint9/LConn1 -- Cartesian Joint8/LConn1
  Graphic3/RConn1 -- Cartesian Joint2/RConn1
  Cartesian Joint/RConn1 -- Graphic1/RConn1
  Graphic4/RConn1 -- Cartesian Joint3/RConn1
  Simulink-PS Converter19/RConn1 -- Cartesian Joint/LConn4

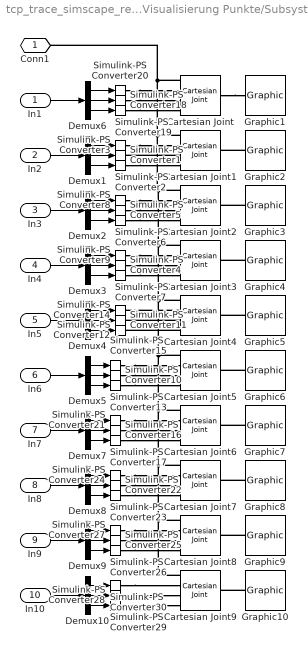
== system tcp_trace_simscape_ref_subsys/Visualisierung Punkte/Subsystem6 ==
  In1 : Inport
  In2 : Inport  Port=2
  In3 : Inport  Port=3
  In4 : Inport  Port=4
  In5 : Inport  Port=5
  In6 : Inport  Port=6
  In7 : Inport  Port=7
  In8 : Inport  Port=8
  In9 : Inport  Port=9
  In10 : Inport  Port=10
  Cartesian Joint{,1..9} (10 alike) : sm_lib/Joints/Cartesian Joint  JointMode=Normal  SenseConstraintForce=off  SenseConstraintForceX=off  SenseConstraintForceY=off  SenseConstraintForceZ=off  SenseConstraintTorque=off  SenseConstraintTorqueX=off  SenseConstraintTorqueY=off  SenseConstraintTorqueZ=off  SenseTotalForce=off  SenseTotalForceX=off  SenseTotalForceY=off  SenseTotalForceZ=off  SenseTotalTorque=off  SenseTotalTorqueX=off  SenseTotalTorqueY=off  SenseTotalTorqueZ=off  CompositeWrenchDir=FollowerOnBase  CompositeWrenchFrame=BaseFrame  PxEquilibriumPosition=0  PxEquilibriumPositionUnits=m  PxSpringStiffness=0  PxSpringStiffnessUnits=N/m  PxDampingCoefficient=0  PxDampingCoefficientUnits=N/(m/s)  PxTorqueActuationMode=ComputedTorque  PxMotionActuationMode=InputMotion  PxSensePosition=off  PxSenseVelocity=off  PxSenseAcceleration=off  PxSenseTorqueForce=off  PxSenseLowerLimitTorqueForce=off  PxSenseUpperLimitTorqueForce=off  PxLowerLimitSpecify=off  PxLowerLimitBound=-1  PxLowerLimitBoundUnits=m  PxLowerLimitStiffness=1e6  PxLowerLimitStiffnessUnits=N/m  PxLowerLimitDamping=1e3  PxLowerLimitDampingUnits=N/(m/s)  PxLowerLimitTransitionRegionWidth=1e-4  PxLowerLimitTransitionRegionWidthUnits=m  PxUpperLimitSpecify=off  PxUpperLimitBound=1  PxUpperLimitBoundUnits=m  PxUpperLimitStiffness=1e6  PxUpperLimitStiffnessUnits=N/m  PxUpperLimitDamping=1e3  PxUpperLimitDampingUnits=N/(m/s)  PxUpperLimitTransitionRegionWidth=1e-4  PxUpperLimitTransitionRegionWidthUnits=m  PxPositionTargetSpecify=off  PxPositionTargetPriority=High  PxPositionTargetValue=0  PxPositionTargetValueUnits=m  PxVelocityTargetSpecify=off  PxVelocityTargetPriority=High  PxVelocityTargetValue=0  PxVelocityTargetValueUnits=m/s  PyEquilibriumPosition=0  PyEquilibriumPositionUnits=m  PySpringStiffness=0  PySpringStiffnessUnits=N/m  PyDampingCoefficient=0  PyDampingCoefficientUnits=N/(m/s)  PyTorqueActuationMode=ComputedTorque  PyMotionActuationMode=InputMotion  PySensePosition=off  PySenseVelocity=off  PySenseAcceleration=off  PySenseTorqueForce=off  PySenseLowerLimitTorqueForce=off  PySenseUpperLimitTorqueForce=off  PyLowerLimitSpecify=off  PyLowerLimitBound=-1  PyLowerLimitBoundUnits=m  PyLowerLimitStiffness=1e6  PyLowerLimitStiffnessUnits=N/m  PyLowerLimitDamping=1e3  PyLowerLimitDampingUnits=N/(m/s)  PyLowerLimitTransitionRegionWidth=1e-4  PyLowerLimitTransitionRegionWidthUnits=m  PyUpperLimitSpecify=off  PyUpperLimitBound=1  PyUpperLimitBoundUnits=m  PyUpperLimitStiffness=1e6  PyUpperLimitStiffnessUnits=N/m  PyUpperLimitDamping=1e3  PyUpperLimitDampingUnits=N/(m/s)  PyUpperLimitTransitionRegionWidth=1e-4  PyUpperLimitTransitionRegionWidthUnits=m  PyPositionTargetSpecify=off  PyPositionTargetPriority=High  PyPositionTargetValue=0  PyPositionTargetValueUnits=m  PyVelocityTargetSpecify=off  PyVelocityTargetPriority=High  PyVelocityTargetValue=0  PyVelocityTargetValueUnits=m/s  PzEquilibriumPosition=0  PzEquilibriumPositionUnits=m  PzSpringStiffness=0  PzSpringStiffnessUnits=N/m  PzDampingCoefficient=0  PzDampingCoefficientUnits=N/(m/s)  PzTorqueActuationMode=ComputedTorque  PzMotionActuationMode=InputMotion  PzSensePosition=off  PzSenseVelocity=off  PzSenseAcceleration=off  PzSenseTorqueForce=off  PzSenseLowerLimitTorqueForce=off  PzSenseUpperLimitTorqueForce=off  PzLowerLimitSpecify=off  PzLowerLimitBound=-1  PzLowerLimitBoundUnits=m  PzLowerLimitStiffness=1e6  PzLowerLimitStiffnessUnits=N/m  PzLowerLimitDamping=1e3  PzLowerLimitDampingUnits=N/(m/s)  PzLowerLimitTransitionRegionWidth=1e-4  PzLowerLimitTransitionRegionWidthUnits=m  PzUpperLimitSpecify=off  PzUpperLimitBound=1  PzUpperLimitBoundUnits=m  PzUpperLimitStiffness=1e6  PzUpperLimitStiffnessUnits=N/m  PzUpperLimitDamping=1e3  PzUpperLimitDampingUnits=N/(m/s)  PzUpperLimitTransitionRegionWidth=1e-4  PzUpperLimitTransitionRegionWidthUnits=m  PzPositionTargetSpecify=off  PzPositionTargetPriority=High  PzPositionTargetValue=0  PzPositionTargetValueUnits=m  PzVelocityTargetSpecify=off  PzVelocityTargetPriority=High  PzVelocityTargetValue=0  PzVelocityTargetValueUnits=m/s
  Demux{1..10} (10 alike) : Demux  Outputs=3
  Graphic{1..10} (10 alike) : sm_lib/Body Elements/Graphic  GraphicType=Marker  MarkerShape=Sphere  MarkerSize=param_vis.vis_point.pix  GraphicVisPropType=SimpleVisualProperties  GraphicDiffuseColor=param_vis.vis_point.col  GraphicSpecularColor=[0.5 0.5 0.5 1.0]  GraphicAmbientColor=[0.15 0.15 0.15 1.0]  GraphicEmissiveColor=[0.0 0.0 0.0 1.0]  GraphicShininess=75  GraphicOpacity=param_vis.vis_point.opa
  Simulink-PS Converter{1..30} (30 alike) : nesl_utility/Simulink-PS Converter  PhysicalDomain=network_engine_domain  SubClassName=ps_input  LeftPortType=input  RightPortType=output  PseudoPeriodic=off  Frequencies=[]  NoiseDistribution=none  NoiseParameters=[]  Unit=1  AffineConversion=off  FilteringAndDerivatives=zero  SimscapeFilterOrder=2  InputFilterTimeConstant=0.001  UdotUserProvided=0
  Conn1 : PMIOPort  Side=Left
  wires:
  In7/1 -> Demux7/1
  In6/1 -> Demux5/1
  In10/1 -> Demux10/1
  In2/1 -> Demux1/1
  In5/1 -> Demux4/1
  In4/1 -> Demux3/1
  Demux6/3 -> Simulink-PS Converter19/1
  In3/1 -> Demux2/1
  In1/1 -> Demux6/1
  In9/1 -> Demux9/1
  In8/1 -> Demux8/1
  Demux6/1 -> Simulink-PS Converter20/1
  Demux6/2 -> Simulink-PS Converter18/1
  Demux1/1 -> Simulink-PS Converter3/1
  Demux4/2 -> Simulink-PS Converter11/1
  Demux4/1 -> Simulink-PS Converter14/1
  Demux4/3 -> Simulink-PS Converter12/1
  Demux1/2 -> Simulink-PS Converter1/1
  Demux1/3 -> Simulink-PS Converter2/1
  Demux2/1 -> Simulink-PS Converter8/1
  Demux2/2 -> Simulink-PS Converter5/1
  Demux2/3 -> Simulink-PS Converter6/1
  Demux3/3 -> Simulink-PS Converter7/1
  Demux3/1 -> Simulink-PS Converter9/1
  Demux3/2 -> Simulink-PS Converter4/1
  Demux5/1 -> Simulink-PS Converter15/1
  Demux5/2 -> Simulink-PS Converter10/1
  Demux5/3 -> Simulink-PS Converter13/1
  Demux7/1 -> Simulink-PS Converter21/1
  Demux7/2 -> Simulink-PS Converter16/1
  Demux7/3 -> Simulink-PS Converter17/1
  Demux8/1 -> Simulink-PS Converter24/1
  Demux8/2 -> Simulink-PS Converter22/1
  Demux8/3 -> Simulink-PS Converter23/1
  Demux9/1 -> Simulink-PS Converter27/1
  Demux9/2 -> Simulink-PS Converter25/1
  Demux9/3 -> Simulink-PS Converter26/1
  Demux10/1 -> Simulink-PS Converter30/1
  Demux10/2 -> Simulink-PS Converter28/1
  Demux10/3 -> Simulink-PS Converter29/1
  connections:
  Simulink-PS Converter19/RConn1 -- Cartesian Joint/LConn4
  Graphic4/RConn1 -- Cartesian Joint3/RConn1
  Cartesian Joint/RConn1 -- Graphic1/RConn1
  Graphic3/RConn1 -- Cartesian Joint2/RConn1
  Cartesian Joint8/LConn1 -- Cartesian Joint9/LConn1 -- Cartesian Joint7/LConn1 -- Cartesian Joint6/LConn1 -- Cartesian Joint5/LConn1 -- Cartesian Joint4/LConn1 -- Cartesian Joint3/LConn1 -- Cartesian Joint2/LConn1 -- Cartesian Joint1/LConn1 -- Cartesian Joint/LConn1 -- Conn1/RConn1
  Graphic7/RConn1 -- Cartesian Joint6/RConn1
  Graphic8/RConn1 -- Cartesian Joint7/RConn1
  Graphic6/RConn1 -- Cartesian Joint5/RConn1
  Graphic9/RConn1 -- Cartesian Joint8/RConn1
  Graphic2/RConn1 -- Cartesian Joint1/RConn1
  Graphic5/RConn1 -- Cartesian Joint4/RConn1
  Graphic10/RConn1 -- Cartesian Joint9/RConn1
  Simulink-PS Converter18/RConn1 -- Cartesian Joint/LConn3
  Simulink-PS Converter20/RConn1 -- Cartesian Joint/LConn2
  Simulink-PS Converter6/RConn1 -- Cartesian Joint2/LConn4
  Simulink-PS Converter8/RConn1 -- Cartesian Joint2/LConn2
  Simulink-PS Converter5/RConn1 -- Cartesian Joint2/LConn3
  Cartesian Joint4/LConn4 -- Simulink-PS Converter12/RConn1
  Cartesian Joint4/LConn2 -- Simulink-PS Converter14/RConn1
  Cartesian Joint4/LConn3 -- Simulink-PS Converter11/RConn1
  Simulink-PS Converter3/RConn1 -- Cartesian Joint1/LConn2
  Cartesian Joint1/LConn3 -- Simulink-PS Converter1/RConn1
  Simulink-PS Converter2/RConn1 -- Cartesian Joint1/LConn4
  Simulink-PS Converter15/RConn1 -- Cartesian Joint5/LConn2
  Simulink-PS Converter10/RConn1 -- Cartesian Joint5/LConn3
  Simulink-PS Converter13/RConn1 -- Cartesian Joint5/LConn4
  Simulink-PS Converter21/RConn1 -- Cartesian Joint6/LConn2
  Simulink-PS Converter16/RConn1 -- Cartesian Joint6/LConn3
  Simulink-PS Converter17/RConn1 -- Cartesian Joint6/LConn4
  Simulink-PS Converter24/RConn1 -- Cartesian Joint7/LConn2
  Simulink-PS Converter22/RConn1 -- Cartesian Joint7/LConn3
  Simulink-PS Converter23/RConn1 -- Cartesian Joint7/LConn4
  Simulink-PS Converter27/RConn1 -- Cartesian Joint8/LConn2
  Simulink-PS Converter25/RConn1 -- Cartesian Joint8/LConn3
  Simulink-PS Converter26/RConn1 -- Cartesian Joint8/LConn4
  Simulink-PS Converter30/RConn1 -- Cartesian Joint9/LConn2
  Simulink-PS Converter28/RConn1 -- Cartesian Joint9/LConn3
  Simulink-PS Converter29/RConn1 -- Cartesian Joint9/LConn4
  Simulink-PS Converter9/RConn1 -- Cartesian Joint3/LConn2
  Simulink-PS Converter4/RConn1 -- Cartesian Joint3/LConn3
  Simulink-PS Converter7/RConn1 -- Cartesian Joint3/LConn4

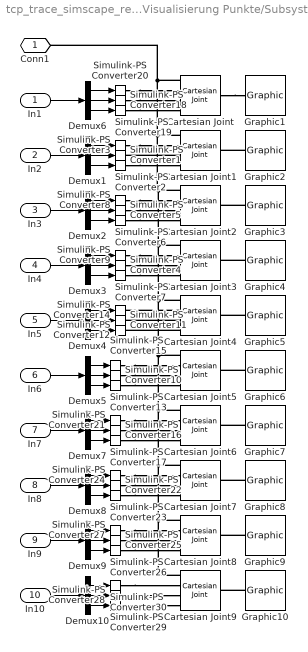
== system tcp_trace_simscape_ref_subsys/Visualisierung Punkte/Subsystem7 ==
  In1 : Inport
  In2 : Inport  Port=2
  In3 : Inport  Port=3
  In4 : Inport  Port=4
  In5 : Inport  Port=5
  In6 : Inport  Port=6
  In7 : Inport  Port=7
  In8 : Inport  Port=8
  In9 : Inport  Port=9
  In10 : Inport  Port=10
  Cartesian Joint{,1..9} (10 alike) : sm_lib/Joints/Cartesian Joint  JointMode=Normal  SenseConstraintForce=off  SenseConstraintForceX=off  SenseConstraintForceY=off  SenseConstraintForceZ=off  SenseConstraintTorque=off  SenseConstraintTorqueX=off  SenseConstraintTorqueY=off  SenseConstraintTorqueZ=off  SenseTotalForce=off  SenseTotalForceX=off  SenseTotalForceY=off  SenseTotalForceZ=off  SenseTotalTorque=off  SenseTotalTorqueX=off  SenseTotalTorqueY=off  SenseTotalTorqueZ=off  CompositeWrenchDir=FollowerOnBase  CompositeWrenchFrame=BaseFrame  PxEquilibriumPosition=0  PxEquilibriumPositionUnits=m  PxSpringStiffness=0  PxSpringStiffnessUnits=N/m  PxDampingCoefficient=0  PxDampingCoefficientUnits=N/(m/s)  PxTorqueActuationMode=ComputedTorque  PxMotionActuationMode=InputMotion  PxSensePosition=off  PxSenseVelocity=off  PxSenseAcceleration=off  PxSenseTorqueForce=off  PxSenseLowerLimitTorqueForce=off  PxSenseUpperLimitTorqueForce=off  PxLowerLimitSpecify=off  PxLowerLimitBound=-1  PxLowerLimitBoundUnits=m  PxLowerLimitStiffness=1e6  PxLowerLimitStiffnessUnits=N/m  PxLowerLimitDamping=1e3  PxLowerLimitDampingUnits=N/(m/s)  PxLowerLimitTransitionRegionWidth=1e-4  PxLowerLimitTransitionRegionWidthUnits=m  PxUpperLimitSpecify=off  PxUpperLimitBound=1  PxUpperLimitBoundUnits=m  PxUpperLimitStiffness=1e6  PxUpperLimitStiffnessUnits=N/m  PxUpperLimitDamping=1e3  PxUpperLimitDampingUnits=N/(m/s)  PxUpperLimitTransitionRegionWidth=1e-4  PxUpperLimitTransitionRegionWidthUnits=m  PxPositionTargetSpecify=off  PxPositionTargetPriority=High  PxPositionTargetValue=0  PxPositionTargetValueUnits=m  PxVelocityTargetSpecify=off  PxVelocityTargetPriority=High  PxVelocityTargetValue=0  PxVelocityTargetValueUnits=m/s  PyEquilibriumPosition=0  PyEquilibriumPositionUnits=m  PySpringStiffness=0  PySpringStiffnessUnits=N/m  PyDampingCoefficient=0  PyDampingCoefficientUnits=N/(m/s)  PyTorqueActuationMode=ComputedTorque  PyMotionActuationMode=InputMotion  PySensePosition=off  PySenseVelocity=off  PySenseAcceleration=off  PySenseTorqueForce=off  PySenseLowerLimitTorqueForce=off  PySenseUpperLimitTorqueForce=off  PyLowerLimitSpecify=off  PyLowerLimitBound=-1  PyLowerLimitBoundUnits=m  PyLowerLimitStiffness=1e6  PyLowerLimitStiffnessUnits=N/m  PyLowerLimitDamping=1e3  PyLowerLimitDampingUnits=N/(m/s)  PyLowerLimitTransitionRegionWidth=1e-4  PyLowerLimitTransitionRegionWidthUnits=m  PyUpperLimitSpecify=off  PyUpperLimitBound=1  PyUpperLimitBoundUnits=m  PyUpperLimitStiffness=1e6  PyUpperLimitStiffnessUnits=N/m  PyUpperLimitDamping=1e3  PyUpperLimitDampingUnits=N/(m/s)  PyUpperLimitTransitionRegionWidth=1e-4  PyUpperLimitTransitionRegionWidthUnits=m  PyPositionTargetSpecify=off  PyPositionTargetPriority=High  PyPositionTargetValue=0  PyPositionTargetValueUnits=m  PyVelocityTargetSpecify=off  PyVelocityTargetPriority=High  PyVelocityTargetValue=0  PyVelocityTargetValueUnits=m/s  PzEquilibriumPosition=0  PzEquilibriumPositionUnits=m  PzSpringStiffness=0  PzSpringStiffnessUnits=N/m  PzDampingCoefficient=0  PzDampingCoefficientUnits=N/(m/s)  PzTorqueActuationMode=ComputedTorque  PzMotionActuationMode=InputMotion  PzSensePosition=off  PzSenseVelocity=off  PzSenseAcceleration=off  PzSenseTorqueForce=off  PzSenseLowerLimitTorqueForce=off  PzSenseUpperLimitTorqueForce=off  PzLowerLimitSpecify=off  PzLowerLimitBound=-1  PzLowerLimitBoundUnits=m  PzLowerLimitStiffness=1e6  PzLowerLimitStiffnessUnits=N/m  PzLowerLimitDamping=1e3  PzLowerLimitDampingUnits=N/(m/s)  PzLowerLimitTransitionRegionWidth=1e-4  PzLowerLimitTransitionRegionWidthUnits=m  PzUpperLimitSpecify=off  PzUpperLimitBound=1  PzUpperLimitBoundUnits=m  PzUpperLimitStiffness=1e6  PzUpperLimitStiffnessUnits=N/m  PzUpperLimitDamping=1e3  PzUpperLimitDampingUnits=N/(m/s)  PzUpperLimitTransitionRegionWidth=1e-4  PzUpperLimitTransitionRegionWidthUnits=m  PzPositionTargetSpecify=off  PzPositionTargetPriority=High  PzPositionTargetValue=0  PzPositionTargetValueUnits=m  PzVelocityTargetSpecify=off  PzVelocityTargetPriority=High  PzVelocityTargetValue=0  PzVelocityTargetValueUnits=m/s
  Demux{1..10} (10 alike) : Demux  Outputs=3
  Graphic{1..10} (10 alike) : sm_lib/Body Elements/Graphic  GraphicType=Marker  MarkerShape=Sphere  MarkerSize=param_vis.vis_point.pix  GraphicVisPropType=SimpleVisualProperties  GraphicDiffuseColor=param_vis.vis_point.col  GraphicSpecularColor=[0.5 0.5 0.5 1.0]  GraphicAmbientColor=[0.15 0.15 0.15 1.0]  GraphicEmissiveColor=[0.0 0.0 0.0 1.0]  GraphicShininess=75  GraphicOpacity=param_vis.vis_point.opa
  Simulink-PS Converter{1..30} (30 alike) : nesl_utility/Simulink-PS Converter  PhysicalDomain=network_engine_domain  SubClassName=ps_input  LeftPortType=input  RightPortType=output  PseudoPeriodic=off  Frequencies=[]  NoiseDistribution=none  NoiseParameters=[]  Unit=1  AffineConversion=off  FilteringAndDerivatives=zero  SimscapeFilterOrder=2  InputFilterTimeConstant=0.001  UdotUserProvided=0
  Conn1 : PMIOPort  Side=Left
  wires:
  Demux10/3 -> Simulink-PS Converter29/1
  Demux10/2 -> Simulink-PS Converter28/1
  Demux10/1 -> Simulink-PS Converter30/1
  Demux9/3 -> Simulink-PS Converter26/1
  Demux9/2 -> Simulink-PS Converter25/1
  Demux9/1 -> Simulink-PS Converter27/1
  Demux8/3 -> Simulink-PS Converter23/1
  Demux8/2 -> Simulink-PS Converter22/1
  Demux8/1 -> Simulink-PS Converter24/1
  Demux7/3 -> Simulink-PS Converter17/1
  Demux7/2 -> Simulink-PS Converter16/1
  Demux7/1 -> Simulink-PS Converter21/1
  Demux5/3 -> Simulink-PS Converter13/1
  Demux5/2 -> Simulink-PS Converter10/1
  Demux5/1 -> Simulink-PS Converter15/1
  Demux3/2 -> Simulink-PS Converter4/1
  Demux3/1 -> Simulink-PS Converter9/1
  Demux3/3 -> Simulink-PS Converter7/1
  Demux2/3 -> Simulink-PS Converter6/1
  Demux2/2 -> Simulink-PS Converter5/1
  Demux2/1 -> Simulink-PS Converter8/1
  Demux1/3 -> Simulink-PS Converter2/1
  Demux1/2 -> Simulink-PS Converter1/1
  Demux4/3 -> Simulink-PS Converter12/1
  Demux4/1 -> Simulink-PS Converter14/1
  Demux4/2 -> Simulink-PS Converter11/1
  Demux1/1 -> Simulink-PS Converter3/1
  Demux6/2 -> Simulink-PS Converter18/1
  Demux6/1 -> Simulink-PS Converter20/1
  In8/1 -> Demux8/1
  In9/1 -> Demux9/1
  In1/1 -> Demux6/1
  In3/1 -> Demux2/1
  Demux6/3 -> Simulink-PS Converter19/1
  In4/1 -> Demux3/1
  In5/1 -> Demux4/1
  In2/1 -> Demux1/1
  In10/1 -> Demux10/1
  In6/1 -> Demux5/1
  In7/1 -> Demux7/1
  connections:
  Simulink-PS Converter7/RConn1 -- Cartesian Joint3/LConn4
  Simulink-PS Converter4/RConn1 -- Cartesian Joint3/LConn3
  Simulink-PS Converter9/RConn1 -- Cartesian Joint3/LConn2
  Simulink-PS Converter29/RConn1 -- Cartesian Joint9/LConn4
  Simulink-PS Converter28/RConn1 -- Cartesian Joint9/LConn3
  Simulink-PS Converter30/RConn1 -- Cartesian Joint9/LConn2
  Simulink-PS Converter26/RConn1 -- Cartesian Joint8/LConn4
  Simulink-PS Converter25/RConn1 -- Cartesian Joint8/LConn3
  Simulink-PS Converter27/RConn1 -- Cartesian Joint8/LConn2
  Simulink-PS Converter23/RConn1 -- Cartesian Joint7/LConn4
  Simulink-PS Converter22/RConn1 -- Cartesian Joint7/LConn3
  Simulink-PS Converter24/RConn1 -- Cartesian Joint7/LConn2
  Simulink-PS Converter17/RConn1 -- Cartesian Joint6/LConn4
  Simulink-PS Converter16/RConn1 -- Cartesian Joint6/LConn3
  Simulink-PS Converter21/RConn1 -- Cartesian Joint6/LConn2
  Simulink-PS Converter13/RConn1 -- Cartesian Joint5/LConn4
  Simulink-PS Converter10/RConn1 -- Cartesian Joint5/LConn3
  Simulink-PS Converter15/RConn1 -- Cartesian Joint5/LConn2
  Simulink-PS Converter2/RConn1 -- Cartesian Joint1/LConn4
  Cartesian Joint1/LConn3 -- Simulink-PS Converter1/RConn1
  Simulink-PS Converter3/RConn1 -- Cartesian Joint1/LConn2
  Cartesian Joint4/LConn3 -- Simulink-PS Converter11/RConn1
  Cartesian Joint4/LConn2 -- Simulink-PS Converter14/RConn1
  Cartesian Joint4/LConn4 -- Simulink-PS Converter12/RConn1
  Simulink-PS Converter5/RConn1 -- Cartesian Joint2/LConn3
  Simulink-PS Converter8/RConn1 -- Cartesian Joint2/LConn2
  Simulink-PS Converter6/RConn1 -- Cartesian Joint2/LConn4
  Simulink-PS Converter20/RConn1 -- Cartesian Joint/LConn2
  Simulink-PS Converter18/RConn1 -- Cartesian Joint/LConn3
  Graphic10/RConn1 -- Cartesian Joint9/RConn1
  Graphic5/RConn1 -- Cartesian Joint4/RConn1
  Graphic2/RConn1 -- Cartesian Joint1/RConn1
  Graphic9/RConn1 -- Cartesian Joint8/RConn1
  Graphic6/RConn1 -- Cartesian Joint5/RConn1
  Graphic8/RConn1 -- Cartesian Joint7/RConn1
  Graphic7/RConn1 -- Cartesian Joint6/RConn1
  Conn1/RConn1 -- Cartesian Joint/LConn1 -- Cartesian Joint1/LConn1 -- Cartesian Joint2/LConn1 -- Cartesian Joint3/LConn1 -- Cartesian Joint4/LConn1 -- Cartesian Joint5/LConn1 -- Cartesian Joint6/LConn1 -- Cartesian Joint7/LConn1 -- Cartesian Joint9/LConn1 -- Cartesian Joint8/LConn1
  Graphic3/RConn1 -- Cartesian Joint2/RConn1
  Cartesian Joint/RConn1 -- Graphic1/RConn1
  Graphic4/RConn1 -- Cartesian Joint3/RConn1
  Simulink-PS Converter19/RConn1 -- Cartesian Joint/LConn4
